simulink subsystem "DCMotorModel"  (R2023b)
settings: Solver=VariableStepAuto  StartTime=0.0  StopTime=10.0  RelTol=1e-3
model mask{L=570*1e-6, R=22, Kt=3.56*1e-3, B=3.42*(1e-6)/((2*pi/60)*1e3), J=0.5*0.05*(0.05^2)}
values from neighbouring files (symbols this model uses):
  B = 20    [quaternionTest.m]
  R = [1 - 2*(qj^2 + qk^2),  2*(qi*qj - qk*qr),   2*(qi*qk + qj*qr) ... (first row only)    [quat2rotmat.m]
libraries: slpidlib x1
settings Model: Creator=andrea  LastModifiedBy=andrea

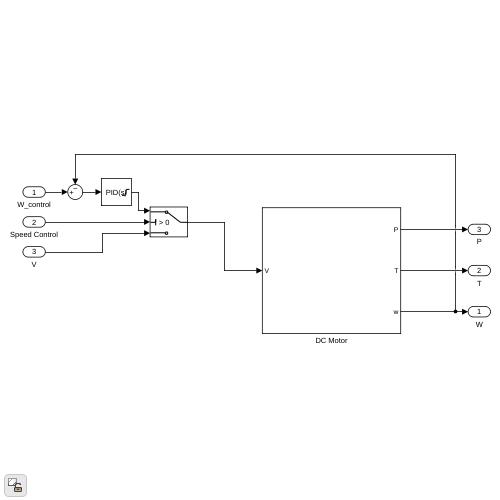
[thumbnail: Simulink's stored preview of the top-level diagram]
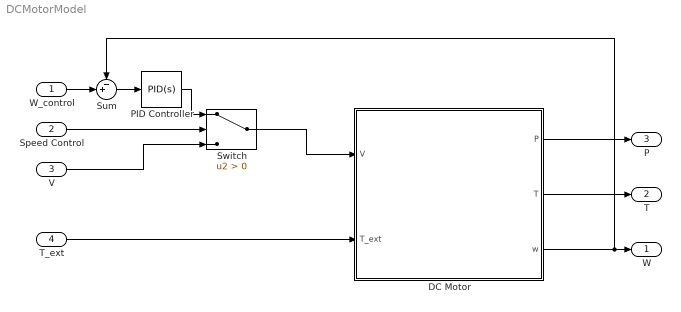
== system DCMotorModel ==
  W_control : Inport
  Speed Control : Inport  Port=2
  V : Inport  Port=3
  T_ext : Inport  Port=4
  DC Motor : Subsystem
  PID Controller : slpidlib/PID Controller  Controller=PID  Form=Parallel  TimeDomain=Continuous-time  UseExternalTs=off  SampleTime=-1  IntegratorMethod=Forward Euler  FilterMethod=Forward Euler  ControllerParametersSource=internal  P=0.0135694485712718  I=0.254571726895349  UseKiTs=off  D=0  N=61.146147680322  UseFilter=on  TunerSelectOption=Transfer Function Based (PID Tuner App)  InitialConditionSource=internal  InitialConditionForIntegrator=0  InitialConditionForFilter=0  DifferentiatorICPrevScaledInput=0  ExternalReset=none  TrackingMode=off  Kt=1  LimitOutput=on  SatLimitsSource=internal  UpperSaturationLimit=6  LowerSaturationLimit=-6  LinearizeAsGain=on  AntiWindupMode=clamping  Kb=1  LimitIntegrator=on  UpperIntegratorSaturationLimit=6  LowerIntegratorSaturationLimit=-6  POutMin=[]  POutMax=[]  IOutMin=[]  IOutMax=[]  DOutMin=[]  DOutMax=[]  NOutMin=[]  NOutMax=[]  SumOutMin=[]  SumOutMax=[]  SaturationOutMin=[]  SaturationOutMax=[]  PParamMin=[]  PParamMax=[]  IParamMin=[]  IParamMax=[]  DParamMin=[]  DParamMax=[]  NParamMin=[]  NParamMax=[]  KbParamMin=[]  KbParamMax=[]  KtParamMin=[]  KtParamMax=[]  KbOutMin=[]  KbOutMax=[]  KtOutMin=[]  KtOutMax=[]  IntegratorOutMin=[]  IntegratorOutMax=[]  FilterOutMin=[]  FilterOutMax=[]  SumI1OutMin=[]  SumI1OutMax=[]  SumI2OutMin=[]  SumI2OutMax=[]  SumI3OutMin=[]  SumI3OutMax=[]  SumI4OutMin=[]  SumI4OutMax=[]  SumDOutMin=[]  SumDOutMax=[]  DifferentiatorOutMin=[]  DifferentiatorOutMax=[]  FilterDiffOutCoefMin=[]  FilterDiffOutCoefMax=[]  ReciprocalOutMin=[]  ReciprocalOutMax=[]  SumDenOutMin=[]  SumDenOutMax=[]  SumNumOutMin=[]  SumNumOutMax=[]  DivideOutMin=[]  DivideOutMax=[]  UdiffTsProdOutMin=[]  UdiffTsProdOutMax=[]  NTsProdOutMin=[]  NTsProdOutMax=[]  UintegralTsProdOutMin=[]  UintegralTsProdOutMax=[]  UngainTsProdOutMin=[]  UngainTsProdOutMax=[]  ClampingZeroOutDataTypeStr=Inherit: Inherit via back propagation  ClampingZeroOutMin=[]  ClampingZeroOutMax=[]  FilterDenConstantOutDataTypeStr=Inherit: Inherit via back propagation  FilterDenConstantOutMin=[]  FilterDenConstantOutMax=[]  PCopyOutDataTypeStr=Inherit: Inherit via back propagation  PCopyOutMin=[]  PCopyOutMax=[]  NCopyOutDataTypeStr=Inherit: Inherit via back propagation  NCopyOutMin=[]  NCopyOutMax=[]  IntegratorContinuousStateAttributes=''  IntegratorStateMustResolveToSignalObject=off  IntegratorRTWStateStorageClass=Auto  FilterContinuousStateAttributes=''  FilterStateMustResolveToSignalObject=off  FilterRTWStateStorageClass=Auto  ParallelPVariant=InternalParameters  IdealPVariant=Disabled  IVariant=InternalParameters  DVariant=InternalParameters  IntegratorVariant=Continuous  SatVariant=Enabled  AWVariant=ContClampingParallel  PCopyVariant=Disabled  TRVariant=Disabled  FdbkBlocksVariant=Forward  IdealPFdbkVariant=Disabled  SatFdbkVariant=Disabled  DerivativeFilterVariant=ContFilter  NVariant=InternalParameters  NCopyVariant=Disabled  FilterICVariant=InternalICsFilter  IntegratorICVariant=InternalICs  ExternalResetVariant=Disabled  TRSumVariant=Passthrough  SumFdbkVariant=Disabled  SumVariant=Sum_PID  TsampFilterVariant=InternalTs  TsampNgainVariant=Passthrough  TsampIntegralVariant=Disabled_SignalSpec  ExternalSaturationOutDataTypeStr=Inherit: Same as second input
  Sum : Sum  Inputs=-+|
  Switch : Switch  Criteria=u2 > Threshold  SaturateOnIntegerOverflow=off  InputSameDT=off
  W : Outport
  T : Outport  Port=2
  P : Outport  Port=3
  wires:
  DC Motor/1(P) -> P/1
  DC Motor/2(T) -> T/1
  Switch/1 -> DC Motor/1(V)
  Sum/1 -> PID Controller/1
  DC Motor/3(w) -> W/1, Sum/1
  W_control/1 -> Sum/2
  PID Controller/1 -> Switch/1
  Speed Control/1 -> Switch/2
  V/1 -> Switch/3
  T_ext/1 -> DC Motor/2(T_ext)

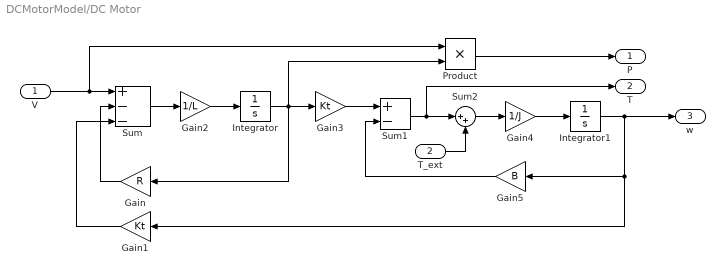
== system DCMotorModel/DC Motor ==
  V : Inport
  T_ext : Inport  Port=2
  Gain : Gain  Gain=R
  Gain1 : Gain  Gain=Kt
  Gain2 : Gain  Gain=1/L
  Gain3 : Gain  Gain=Kt
  Gain4 : Gain  Gain=1/J
  Gain5 : Gain  Gain=B
  Integrator : Integrator
  Integrator1 : Integrator
  Product : Product
  Sum : Sum  Inputs=+--
  Sum1 : Sum  Inputs=+-
  Sum2 : Sum  Inputs=|++
  P : Outport
  T : Outport  Port=2
  w : Outport  Port=3
  wires:
  T_ext/1 -> Sum2/2
  Sum2/1 -> Gain4/1
  Product/1 -> P/1
  Gain5/1 -> Sum1/2
  Integrator1/1 -> w/1, Gain5/1, Gain1/1
  Gain4/1 -> Integrator1/1
  Sum1/1 -> T/1, Sum2/1
  Gain3/1 -> Sum1/1
  Integrator/1 -> Gain/1, Gain3/1, Product/2
  Gain2/1 -> Integrator/1
  Sum/1 -> Gain2/1
  Gain1/1 -> Sum/3
  Gain/1 -> Sum/2
  V/1 -> Sum/1, Product/1
